simulink model "HighLevel_RaspberryPi"  (R2016a)
settings: Solver=ode3  StartTime=0.0  StopTime=inf  RelTol=1e-3
model workspace (MAT data in the model file):
  neighborhood = [301 101]
  num_pics = 16
undefined symbols (not defined in the file): gray
libraries: simulink x21, dspswit3 x6, visiontextngfix x5, visiontransforms x2, embdlinuxlib x2, visionanalysis x1, visionstatistics x1, visiongeotforms x1
settings Model: SimulationMode=external  ExtModeTrigDuration=100  Creator=Grisha  LastModifiedBy=Ryhor
settings SolverCC: PositivePriorityOrder=on
settings DataIOCC: LimitDataPoints=on  SaveOutput=off  SignalLogging=off  SaveTime=off
settings OptimizationCC: EfficientMapNaN2IntZero=off  OptimizeModelRefInitCode=on  LifeSpan=Inf  MaxStackSize=64
settings DebuggingCC: MultiTaskRateTransMsg=warning  ParameterPrecisionLossMsg=none  AllowSymbolicDim=off  StateNameClashWarn=warning
settings HardwareCC: ProdBitPerPointer=32  ProdLargestAtomicInteger=Long  ProdLargestAtomicFloat=Double  ProdWordSize=32  ProdHWDeviceType=ARM Compatible->ARM Cortex
settings ModelReferenceCC: PropagateSignalLabelsOutOfModel=off
settings RTWCC: SystemTargetFile=ert.tlc  HardwareBoard=Raspberry Pi  TemplateMakefile=ert_default_tmf  GenerateReport=on  RTWVerbose=off  Toolchain=GNU GCC Raspberry Pi  IncludeHyperlinkInReport=on  LaunchReport=on  GenerateTraceInfo=on  GenerateTraceReport=on  GenerateTraceReportSl=on  GenerateTraceReportSf=on  GenerateTraceReportEml=on
settings CodeAppCC: ForceParamTrailComments=on  IgnoreCustomStorageClasses=off  OperatorAnnotations=on  SimulinkDataObjDesc=on  SFDataObjDesc=on  MATLABFcnDesc=on  MangleLength=10  InsertBlockDesc=on  MATLABSourceComments=on
settings ERTTargetCC: SupportVariableSizeSignals=on  ExtMode=on  ExtModeMexArgs='192.168.1.102' 0 17725

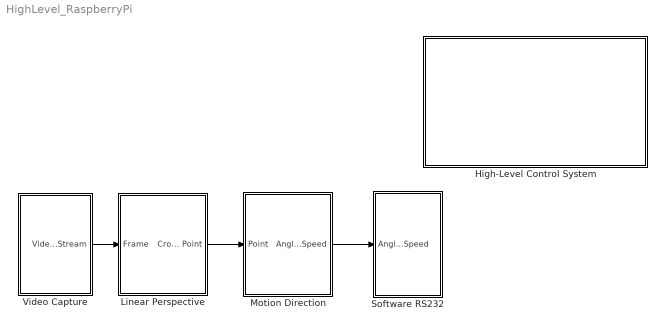
== system HighLevel_RaspberryPi ==
  High-Level Control System : Subsystem
      mask Display: image('C:\Users\Ryhor\Pictures\raspberry-pi-2-primary-100569130-large.png');
  Linear Perspective : Subsystem
  Motion Direction : Subsystem
  Software RS232 : Subsystem
  Video Capture : Subsystem
  wires:
  Motion Direction/1(Angle Speed) -> Software RS232/1(Angle Speed)
  Video Capture/1(Video Stream) -> Linear Perspective/1(Frame)
  Linear Perspective/1(Cross Point) -> Motion Direction/1(Point)

== system HighLevel_RaspberryPi/High-Level Control System ==

== system HighLevel_RaspberryPi/Linear Perspective ==
  Frame : Inport
  Edge Detection : visionanalysis/Edge Detection  method=Roberts  outputType=Binary image  userDefinedThreshold=off  thresholdSource=Input port  threshold=20  thresholdTuning=4  edgeThinning=off  threshold_canny=[0.25 0.60]  autoPercent=90  sigma=1  prodOutputMode=Binary point scaling  prodOutputWordLength=32  prodOutputFracLength=8  roundingMode=Floor  overflowMode=off
  Find Al Lines From HoughTransforms : Subsystem
  Line Sort : Subsystem
  Lines Crossing Points : Subsystem
  Cross Point : Outport
  wires:
  Find Al Lines From HoughTransforms/1(All_Lines) -> Line Sort/2(All Lines)
  Line Sort/2(Desired Line Coord) -> Lines Crossing Points/2(Line Coord)
  Line Sort/1(Image Out) -> Lines Crossing Points/1(Image In)
  Edge Detection/1 -> Find Al Lines From HoughTransforms/1(BW)
  Lines Crossing Points/1(Cross Point) -> Cross Point/1
  Frame/1 -> Find Al Lines From HoughTransforms/2(Grey), Line Sort/1(RGB Image), Edge Detection/1

== system HighLevel_RaspberryPi/Motion Direction ==
  Point : Inport
  Constant : Constant  Value=160  OutDataTypeStr=uint16
  Constant1 : Constant  Value=140  OutDataTypeStr=uint8
  Constant2 : Constant  Value=100  OutDataTypeStr=uint8
  Selector : Selector  NumberOfDimensions=2  InputPortWidth=3  IndexOptions=Index vector (dialog),Index vector (dialog)  Indices=1 ,1  OutputSizes=1,1
  Sum : Sum  Inputs=|+-
  Switch : Switch  Criteria=u2 > Threshold
  Angle Speed : Outport
  wires:
  Constant/1 -> Sum/2
  Constant1/1 -> Switch/1
  Constant2/1 -> Switch/3
  Point/1 -> Selector/1
  Selector/1 -> Sum/1
  Sum/1 -> Switch/2
  Switch/1 -> Angle Speed/1

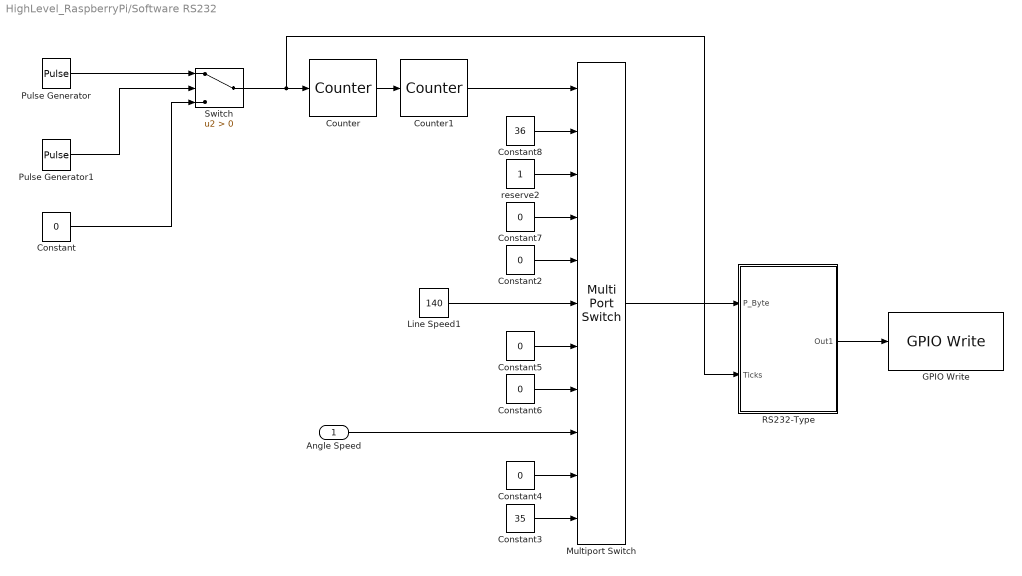
== system HighLevel_RaspberryPi/Software RS232 ==
  Angle Speed : Inport
  Constant : Constant  Value=0  OutDataTypeStr=boolean
  Constant{2,4..7} (5 alike) : Constant  Value=0
  Constant3 : Constant  Value=35
  Constant8 : Constant  Value=36
  Counter : dspswit3/Counter  Direction=Up  CountEvent=Rising edge  CounterSize=User defined  MaxCount=16  InitialCount=1  Output=Hit  HitValue=16  ResetInput=off  SamplesPerFrame=1  Ts=1  CntDtype=double  HitDtype=Logical
  Counter1 : dspswit3/Counter  Direction=Up  CountEvent=Rising edge  CounterSize=User defined  MaxCount=9  InitialCount=0  Output=Count  HitValue=16  ResetInput=off  SamplesPerFrame=1  Ts=1  CntDtype=double  HitDtype=Logical
  GPIO Write : embdlinuxlib/GPIO Write  board=Pi 2 Model B  gpio=14  direction=Output  blockPlatform=Raspberry Pi
  Line Speed1 : Constant  Value=140
  Multiport Switch : MultiPortSwitch  DataPortOrder=Zero-based contiguous  Inputs=10
  Pulse Generator : DiscretePulseGenerator  PulseType=Time based  Period=1/2400  PulseWidth=50  SampleTime=10/57600/16
  Pulse Generator1 : DiscretePulseGenerator  PulseType=Time based  Period=1  PulseWidth=160/2400*100  SampleTime=10/57600/16
  RS232-Type : Subsystem
  Switch : Switch  Criteria=u2 > Threshold
  reserve2 : Constant
  wires:
  Angle Speed/1 -> Multiport Switch/9
  Line Speed1/1 -> Multiport Switch/6
  Constant3/1 -> Multiport Switch/11
  Constant4/1 -> Multiport Switch/10
  Constant6/1 -> Multiport Switch/8
  Constant5/1 -> Multiport Switch/7
  reserve2/1 -> Multiport Switch/3
  Constant8/1 -> Multiport Switch/2
  Constant7/1 -> Multiport Switch/4
  Constant2/1 -> Multiport Switch/5
  Counter/1 -> Counter1/1
  Counter1/1 -> Multiport Switch/1
  Switch/1 -> RS232-Type/2(Ticks), Counter/1
  RS232-Type/1(Out1) -> GPIO Write/1
  Multiport Switch/1 -> RS232-Type/1(P_Byte)
  Pulse Generator/1 -> Switch/1
  Pulse Generator1/1 -> Switch/2
  Constant/1 -> Switch/3

== system HighLevel_RaspberryPi/Video Capture ==
  Rotate : visiongeotforms/Rotate  outSizeR=Expanded to fit rotated input image  src_angle=Specify via dialog  unit_angle=Degrees  angle=pi/2  maxAngle=pi  dispImage=Center  method=Table lookup  fillVal=0  interpMethod=Bilinear  prodOutputMode=Binary point scaling  prodOutputWordLength=32  prodOutputFracLength=10  roundingMode=Nearest  overflowMode=on
  Terminator : Terminator
  Terminator1 : Terminator
  V4L2 Video Capture : embdlinuxlib/V4L2 Video Capture  m_devName='/dev/video0'  roi=[0, 0, 640, 480]  imSizeSelection=320x240  imSize=[640, 480]  pixelFormat=YCbCr 4:2:2  pixelOrder=Planar  sampleTime=1/4  simOutput=Colorbars  blockPlatform=Raspberry Pi
  Video Stream : Outport
  wires:
  V4L2 Video Capture/2 -> Terminator/1
  V4L2 Video Capture/1 -> Rotate/1
  V4L2 Video Capture/3 -> Terminator1/1
  Rotate/1 -> Video Stream/1

== system HighLevel_RaspberryPi/Linear Perspective/Find Al Lines From HoughTransforms ==
  BW : Inport
  Grey : Inport  Port=2
  Constant : Constant  Value=1000
  Find Local Maxima1 : visionstatistics/Find Local Maxima  num_peaks=num_pics  nhood_size=[21 21]  src_thresh=Obsolete9b  src_thresh_inuse=Input port  threshold=1  inputIsHough=on  dt_peak=uint16  isOutVarDim=on  dt_count=uint16
  Find_All_Lines : Subsystem
  Hough Transform : visiontransforms/Hough Transform  theta_res=pi/180  rho_res=1  out_theta_rho=on  outdtmode=double  firstCoeffMode=Binary point scaling  firstCoeffWordLength=16  firstCoeffFracLength=14  secondCoeffMode=Binary point scaling  secondCoeffWordLength=32  secondCoeffFracLength=16  outputMode=Binary point scaling  outputWordLength=16  outputFracLength=0  accumMode=Binary point scaling  accumWordLength=32  accumFracLength=20  prodOutputMode=Binary point scaling  prodOutputWordLength=32  prodOutputFracLength=20  memoryMode=Binary point scaling  memoryWordLength=32  memoryFracLength=16  roundingMode=Nearest  overflowMode=on
  Slider Gain : simulink/Math Operations/Slider Gain  low=0  gain=0.046083  high=1
  All_Lines : Outport
  wires:
  Find Local Maxima1/1 -> Find_All_Lines/1(In1)
  Hough Transform/3 -> Find_All_Lines/3(Rho)
  Find_All_Lines/1(Out1) -> All_Lines/1
  Hough Transform/1 -> Find Local Maxima1/1
  Slider Gain/1 -> Find Local Maxima1/2
  Grey/1 -> Find_All_Lines/4(Grey)
  Constant/1 -> Slider Gain/1
  Hough Transform/2 -> Find_All_Lines/2(Theta)
  BW/1 -> Hough Transform/1

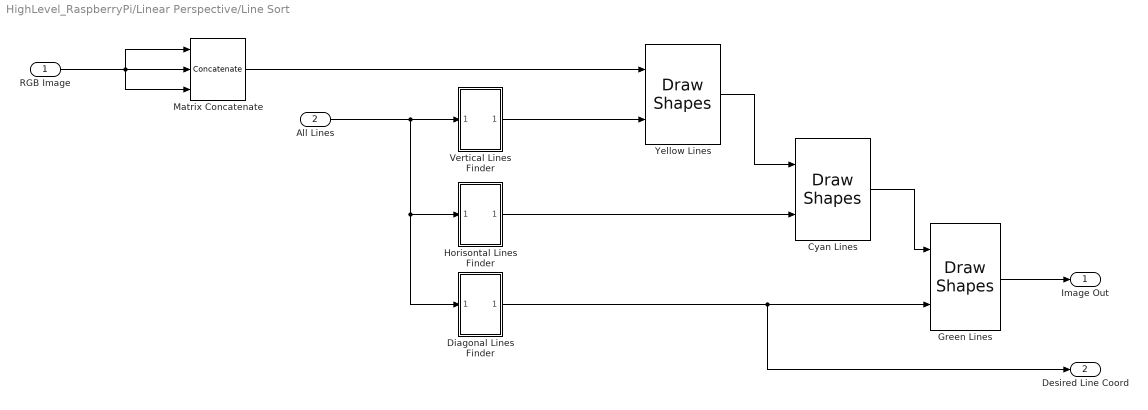
== system HighLevel_RaspberryPi/Linear Perspective/Line Sort ==
  RGB Image : Inport
  All Lines : Inport  Port=2
  Cyan Lines : visiontextngfix/Draw Shapes  shape=Lines  fill=off  lineWidth=2  fillClrSource=Specify via dialog  display=User-specified value  intensity=200  color=[0 100 100]  opacity=0.6  viewport=Entire image  antialiasing=off  inType=Obsolete  imagePorts=One multidimensional signal  prodOutputMode=Binary point scaling  prodOutputWordLength=32  prodOutputFracLength=14  memoryMode=Specify word length  memoryWordLength=16  memoryFracLength=14  roundingMode=Floor  overflowMode=off
  Diagonal Lines Finder : Subsystem
  Green Lines : visiontextngfix/Draw Shapes  shape=Lines  fill=off  lineWidth=1  fillClrSource=Specify via dialog  display=User-specified value  intensity=200  color=[0 255 0]  opacity=0.6  viewport=Entire image  antialiasing=off  inType=Obsolete  imagePorts=One multidimensional signal  prodOutputMode=Binary point scaling  prodOutputWordLength=32  prodOutputFracLength=14  memoryMode=Specify word length  memoryWordLength=16  memoryFracLength=14  roundingMode=Floor  overflowMode=off
  Horisontal Lines Finder : Subsystem
  Matrix Concatenate : Concatenate  NumInputs=3  Mode=Multidimensional array  ConcatenateDimension=3
  Vertical Lines Finder : Subsystem
  Yellow Lines : visiontextngfix/Draw Shapes  shape=Lines  fill=off  lineWidth=2  fillClrSource=Specify via dialog  display=User-specified value  intensity=200  color=[255 255 0]  opacity=0.6  viewport=Entire image  antialiasing=off  inType=Obsolete  imagePorts=One multidimensional signal  prodOutputMode=Binary point scaling  prodOutputWordLength=32  prodOutputFracLength=14  memoryMode=Specify word length  memoryWordLength=16  memoryFracLength=14  roundingMode=Floor  overflowMode=off
  Image Out : Outport
  Desired Line Coord : Outport  Port=2
  wires:
  Vertical Lines Finder/1(Out1) -> Yellow Lines/2
  Cyan Lines/1 -> Green Lines/1
  Diagonal Lines Finder/1(Out2) -> Desired Line Coord/1, Green Lines/2
  Yellow Lines/1 -> Cyan Lines/1
  Horisontal Lines Finder/1(Out1) -> Cyan Lines/2
  Green Lines/1 -> Image Out/1
  All Lines/1 -> Diagonal Lines Finder/1(In1), Horisontal Lines Finder/1(In1), Vertical Lines Finder/1(In1)
  Matrix Concatenate/1 -> Yellow Lines/1
  RGB Image/1 -> Matrix Concatenate/3, Matrix Concatenate/2, Matrix Concatenate/1

== system HighLevel_RaspberryPi/Linear Perspective/Lines Crossing Points ==
  Image In : Inport
  Line Coord : Inport  Port=2
  If : If  IfExpression=u1 > 1
  If Action Subsystem : Subsystem  TreatAsAtomicUnit=on
  If Action Subsystem1 : Subsystem  TreatAsAtomicUnit=on
  Probe : Probe  ProbeWidth=off  ProbeSampleTime=off  ProbeComplexSignal=off  ProbeSignalDimensions=on
  Selector : Selector  NumberOfDimensions=2  InputPortWidth=3  IndexOptions=Index vector (dialog),Index vector (dialog)  Indices=1,1  OutputSizes=1,1
  Switch : Switch  Criteria=u2 > Threshold  Threshold=1
  Video Viewer2 : VideoViewer  colormapValue=gray(256)  FigPos=[716 982 712 582]
  Cross Point : Outport
  wires:
  Probe/1 -> Selector/1
  Selector/1 -> Switch/2, If Action Subsystem/1(In4), If/1
  If/2 -> If Action Subsystem1/Action
  If/1 -> If Action Subsystem/Action
  If Action Subsystem/1(Image Out) -> Switch/1
  If Action Subsystem1/1(Out1) -> Switch/3
  Line Coord/1 -> If Action Subsystem/2(Data Lines), Probe/1
  Image In/1 -> If Action Subsystem1/1(Image In), If Action Subsystem/3(Image In)
  Switch/1 -> Video Viewer2/1
  If Action Subsystem/2(Cross) -> Cross Point/1

== system HighLevel_RaspberryPi/Software RS232/RS232-Type ==
  P_Byte : Inport
  Ticks : Inport  Port=2
  1 + 1+1+ Start Bit : Constant  Value=[1 1 1 0]  OutDataTypeStr=boolean
  Data Type Conv : DataTypeConversion  OutDataTypeStr=boolean
  MATLAB Function : MATLAB Function  TreatAsAtomicUnit=on
  Mux : Mux  Inputs=3
  Parallel-Serial Register 16-1 : Subsystem
  Scope : Scope  NumInputPorts=2
  Stop Bi + 1 + 1 + 1 : Constant  Value=[1 1 1 1]  OutDataTypeStr=boolean
  Out1 : Outport
  wires:
  Parallel-Serial Register 16-1/1(SWord) -> Out1/1, Scope/2
  Mux/1 -> Parallel-Serial Register 16-1/1(P_D_Word)
  Data Type Conv/1 -> Mux/2
  P_Byte/1 -> MATLAB Function/1(u)
  MATLAB Function/1(y) -> Data Type Conv/1
  Ticks/1 -> Scope/1, Parallel-Serial Register 16-1/2(Ticks)
  1 + 1+1+ Start Bit/1 -> Mux/1
  Stop Bi + 1 + 1 + 1/1 -> Mux/3

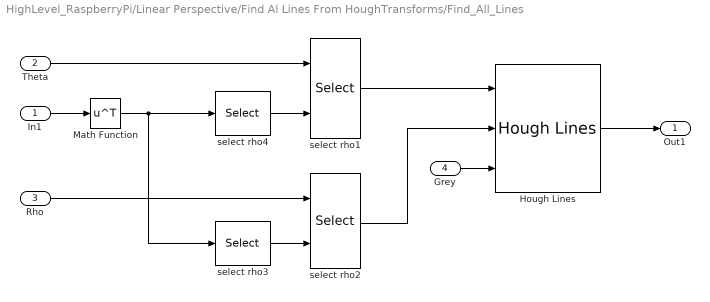
== system HighLevel_RaspberryPi/Linear Perspective/Find Al Lines From HoughTransforms/Find_All_Lines ==
  In1 : Inport
  Theta : Inport  Port=2
  Rho : Inport  Port=3
  Grey : Inport  Port=4
  Hough Lines : visiontransforms/Hough Lines  sineCompMethod=Trigonometric function  thetaRes=pi/180  firstCoeffMode=Specify word length  firstCoeffWordLength=16  firstCoeffFracLength=15  prodOutputMode=Binary point scaling  prodOutputWordLength=32  prodOutputFracLength=16  roundingMode=Nearest  overflowMode=on
  Math Function : Math  Operator=transpose  SaturateOnIntegerOverflow=on
  select rho1 : Selector  NumberOfDimensions=2  InputPortWidth=3  IndexOptions=Select all,Index vector (port)  Indices=1,1  OutputSizes=1,
  select rho2 : Selector  NumberOfDimensions=2  InputPortWidth=3  IndexOptions=Select all,Index vector (port)  Indices=1,1  OutputSizes=1,
  select rho3 : Selector  NumberOfDimensions=2  InputPortWidth=3  IndexOptions=Index vector (dialog),Select all  Indices=2,1  OutputSizes=1,
  select rho4 : Selector  NumberOfDimensions=2  InputPortWidth=3  IndexOptions=Index vector (dialog),Select all  Indices=1,1  OutputSizes=1,
  Out1 : Outport
  wires:
  Theta/1 -> select rho1/1
  Grey/1 -> Hough Lines/3
  In1/1 -> Math Function/1
  select rho2/1 -> Hough Lines/2
  select rho4/1 -> select rho1/2
  select rho3/1 -> select rho2/2
  Rho/1 -> select rho2/1
  Math Function/1 -> select rho3/1, select rho4/1
  Hough Lines/1 -> Out1/1
  select rho1/1 -> Hough Lines/1

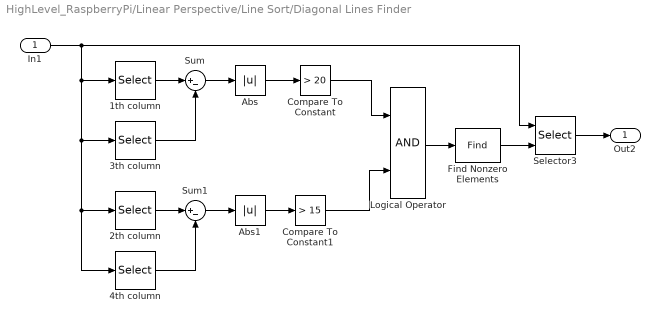
== system HighLevel_RaspberryPi/Linear Perspective/Line Sort/Diagonal Lines Finder ==
  In1 : Inport
  1th column : Selector  NumberOfDimensions=2  InputPortWidth=3  IndexOptions=Select all,Index vector (dialog)  Indices=[1 3],1  OutputSizes=1,1
  2th column : Selector  NumberOfDimensions=2  InputPortWidth=3  IndexOptions=Select all,Index vector (dialog)  Indices=[1 3],2  OutputSizes=1,1
  3th column : Selector  NumberOfDimensions=2  InputPortWidth=3  IndexOptions=Select all,Index vector (dialog)  Indices=[1 3],3  OutputSizes=1,1
  4th column : Selector  NumberOfDimensions=2  InputPortWidth=3  IndexOptions=Select all,Index vector (dialog)  Indices=[1 3],4  OutputSizes=1,1
  Abs : Abs
  Abs1 : Abs
  Compare To Constant : simulink/Logic and Bit Operations/Compare To Constant  relop=>  const=20  OutDataTypeStr=boolean
  Compare To Constant1 : simulink/Logic and Bit Operations/Compare To Constant  relop=>  const=15  OutDataTypeStr=boolean
  Find Nonzero Elements : Find  NumberOfInputDimensions=3
  Logical Operator : Logic  AllPortsSameDT=off  OutDataTypeStr=boolean
  Selector3 : Selector  NumberOfDimensions=2  InputPortWidth=3  IndexOptions=Index vector (port),Select all  Indices=[1 3],3  OutputSizes=1,1
  Sum : Sum  Inputs=|+-
  Sum1 : Sum  Inputs=|+-
  Out2 : Outport
  wires:
  1th column/1 -> Sum/1
  3th column/1 -> Sum/2
  Abs/1 -> Compare To Constant/1
  Sum/1 -> Abs/1
  2th column/1 -> Sum1/1
  4th column/1 -> Sum1/2
  Abs1/1 -> Compare To Constant1/1
  Sum1/1 -> Abs1/1
  Selector3/1 -> Out2/1
  Compare To Constant1/1 -> Logical Operator/2
  In1/1 -> 4th column/1, 2th column/1, 3th column/1, 1th column/1, Selector3/1
  Logical Operator/1 -> Find Nonzero Elements/1
  Compare To Constant/1 -> Logical Operator/1
  Find Nonzero Elements/1 -> Selector3/2

== system HighLevel_RaspberryPi/Linear Perspective/Line Sort/Horisontal Lines Finder ==
  In1 : Inport
  2th column : Selector  NumberOfDimensions=2  InputPortWidth=3  IndexOptions=Select all,Index vector (dialog)  Indices=[1 3],2  OutputSizes=1,1
  4th column : Selector  NumberOfDimensions=2  InputPortWidth=3  IndexOptions=Select all,Index vector (dialog)  Indices=[1 3],4  OutputSizes=1,1
  Abs : Abs
  Compare To Constant : simulink/Logic and Bit Operations/Compare To Constant  relop=<=  const=15  OutDataTypeStr=boolean
  Find Nonzero Elements : Find  NumberOfInputDimensions=3
  Selector3 : Selector  NumberOfDimensions=2  InputPortWidth=3  IndexOptions=Index vector (port),Select all  Indices=[1 3],3  OutputSizes=1,1
  Sum : Sum  Inputs=|+-
  Out1 : Outport
  wires:
  2th column/1 -> Sum/1
  4th column/1 -> Sum/2
  Abs/1 -> Compare To Constant/1
  Sum/1 -> Abs/1
  Selector3/1 -> Out1/1
  Compare To Constant/1 -> Find Nonzero Elements/1
  Find Nonzero Elements/1 -> Selector3/2
  In1/1 -> 4th column/1, 2th column/1, Selector3/1

== system HighLevel_RaspberryPi/Linear Perspective/Line Sort/Vertical Lines Finder ==
  In1 : Inport
  1th column : Selector  NumberOfDimensions=2  InputPortWidth=3  IndexOptions=Select all,Index vector (dialog)  Indices=[1 3],1  OutputSizes=1,1
  3th column : Selector  NumberOfDimensions=2  InputPortWidth=3  IndexOptions=Select all,Index vector (dialog)  Indices=[1 3],3  OutputSizes=1,1
  Abs : Abs
  Compare To Constant : simulink/Logic and Bit Operations/Compare To Constant  relop=<=  const=20  OutDataTypeStr=boolean
  Find Nonzero Elements : Find  NumberOfInputDimensions=3
  Selector3 : Selector  NumberOfDimensions=2  InputPortWidth=3  IndexOptions=Index vector (port),Select all  Indices=[1 3],3  OutputSizes=1,1
  Sum : Sum  Inputs=|+-
  Out1 : Outport
  wires:
  1th column/1 -> Sum/1
  3th column/1 -> Sum/2
  Abs/1 -> Compare To Constant/1
  Sum/1 -> Abs/1
  Selector3/1 -> Out1/1
  Compare To Constant/1 -> Find Nonzero Elements/1
  Find Nonzero Elements/1 -> Selector3/2
  In1/1 -> 3th column/1, 1th column/1, Selector3/1

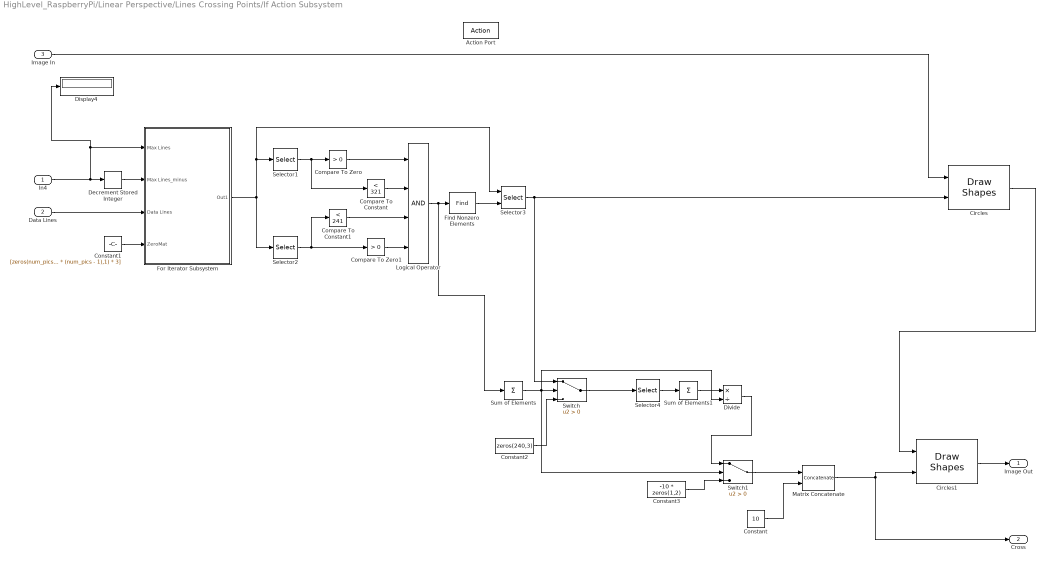
== system HighLevel_RaspberryPi/Linear Perspective/Lines Crossing Points/If Action Subsystem ==
  In4 : Inport
  Data Lines : Inport  Port=2
  Image In : Inport  Port=3
  Action Port : ActionPort  PropagateVarSize=During execution  ActionType=then
  Circles : visiontextngfix/Draw Shapes  shape=Circles  fill=off  lineWidth=2  fillClrSource=Specify via dialog  display=User-specified value  intensity=200  color=[255 0 0]  opacity=0.6  viewport=Entire image  antialiasing=off  inType=Obsolete  imagePorts=One multidimensional signal  prodOutputMode=Binary point scaling  prodOutputWordLength=32  prodOutputFracLength=14  memoryMode=Specify word length  memoryWordLength=16  memoryFracLength=14  roundingMode=Floor  overflowMode=off
  Circles1 : visiontextngfix/Draw Shapes  shape=Circles  fill=off  lineWidth=2  fillClrSource=Specify via dialog  display=User-specified value  intensity=200  color=[200 0 200]  opacity=0.6  viewport=Entire image  antialiasing=off  inType=Obsolete  imagePorts=One multidimensional signal  prodOutputMode=Binary point scaling  prodOutputWordLength=32  prodOutputFracLength=14  memoryMode=Specify word length  memoryWordLength=16  memoryFracLength=14  roundingMode=Floor  overflowMode=off
  Compare To Constant : simulink/Logic and Bit Operations/Compare To Constant  relop=<  const=321  OutDataTypeStr=boolean
  Compare To Constant1 : simulink/Logic and Bit Operations/Compare To Constant  relop=<  const=241  OutDataTypeStr=boolean
  Compare To Zero : simulink/Logic and Bit Operations/Compare To Zero  relop=>  OutDataTypeStr=boolean
  Compare To Zero1 : simulink/Logic and Bit Operations/Compare To Zero  relop=>  OutDataTypeStr=boolean
  Constant : Constant  Value=10  OutDataTypeStr=int32
  Constant1 : Constant  Value=[zeros(num_pics * (num_pics - 1), 2), ones(num_pics * (num_pics - 1),1) * 3]  VectorParams1D=off  OutDataTypeStr=int32
  Constant2 : Constant  Value=zeros(240,3)  VectorParams1D=off  OutDataTypeStr=int32
  Constant3 : Constant  Value=-10 * zeros(1,2)  VectorParams1D=off  OutDataTypeStr=int32
  Decrement Stored Integer : simulink/Additional Math & Discrete/Additional Math: Increment - Decrement/Decrement Stored Integer
  Display4 : Display
  Divide : Product  Inputs=*/
  Find Nonzero Elements : Find  NumberOfInputDimensions=3
  For Iterator Subsystem : Subsystem  TreatAsAtomicUnit=on
  Logical Operator : Logic  Inputs=4  AllPortsSameDT=off  OutDataTypeStr=boolean
  Matrix Concatenate : Concatenate  Mode=Multidimensional array  ConcatenateDimension=2
  Selector1 : Selector  NumberOfDimensions=2  InputPortWidth=3  IndexOptions=Select all,Index vector (dialog)  Indices=[1 3],1  OutputSizes=1,1
  Selector2 : Selector  NumberOfDimensions=2  InputPortWidth=3  IndexOptions=Select all,Index vector (dialog)  Indices=[1 3],2  OutputSizes=1,1
  Selector3 : Selector  NumberOfDimensions=2  InputPortWidth=3  IndexOptions=Index vector (port),Select all  Indices=[1 3],1  OutputSizes=1,1
  Selector4 : Selector  NumberOfDimensions=2  InputPortWidth=3  IndexOptions=Select all,Index vector (dialog)  Indices=[1 3],[1 2]  OutputSizes=1,1
  Sum of Elements : Sum  Inputs=+  AccumDataTypeStr=int32
  Sum of Elements1 : Sum  Inputs=+  CollapseMode=Specified dimension
  Switch : Switch  Criteria=u2 > Threshold
  Switch1 : Switch  Criteria=u2 > Threshold
  Image Out : Outport
  Cross : Outport  Port=2
  wires:
  Find Nonzero Elements/1 -> Selector3/2
  Compare To Zero/1 -> Logical Operator/1
  Compare To Constant1/1 -> Logical Operator/3
  Decrement Stored Integer/1 -> For Iterator Subsystem/2(Max Lines_minus)
  Compare To Constant/1 -> Logical Operator/2
  Selector2/1 -> Compare To Constant1/1, Compare To Zero1/1
  Selector1/1 -> Compare To Zero/1, Compare To Constant/1
  Compare To Zero1/1 -> Logical Operator/4
  For Iterator Subsystem/1(Out1) -> Selector1/1, Selector3/1, Selector2/1
  Logical Operator/1 -> Sum of Elements/1, Find Nonzero Elements/1
  Constant1/1 -> For Iterator Subsystem/4("ZeroMat ")
  In4/1 -> Display4/1, For Iterator Subsystem/1(Max Lines), Decrement Stored Integer/1
  Selector3/1 -> Circles/2, Switch/1
  Data Lines/1 -> For Iterator Subsystem/3(Data Lines)
  Image In/1 -> Circles/1
  Selector4/1 -> Sum of Elements1/1
  Sum of Elements1/1 -> Divide/1
  Divide/1 -> Switch1/1
  Switch/1 -> Selector4/1
  Constant2/1 -> Switch/3
  Constant3/1 -> Switch1/3
  Circles/1 -> Circles1/1
  Matrix Concatenate/1 -> Cross/1, Circles1/2
  Constant/1 -> Matrix Concatenate/2
  Switch1/1 -> Matrix Concatenate/1
  Sum of Elements/1 -> Switch1/2, Divide/2, Switch/2
  Circles1/1 -> Image Out/1

== system HighLevel_RaspberryPi/Linear Perspective/Lines Crossing Points/If Action Subsystem1 ==
  Image In : Inport
  Action Port : ActionPort  ActionType=else
  Out1 : Outport
  wires:
  Image In/1 -> Out1/1

== system HighLevel_RaspberryPi/Software RS232/RS232-Type/Parallel-Serial Register 16-1 ==
  P_D_Word : Inport
  Ticks : Inport  Port=2
  Counter 2^4 : Subsystem
  Demux : Demux  Outputs=8
  Demux1 : Demux  Outputs=8
  High Byte : Selector  InputPortWidth=16  IndexOptions=Index vector (dialog)  Indices=[9:16]  OutputSizes=1
  Low Byte : Selector  InputPortWidth=16  IndexOptions=Index vector (dialog)  Indices=[1:8]  OutputSizes=1
  Multyplexer 8-1 : Subsystem
  Multyplexer 8-2 : Subsystem
  Switch : Switch  Criteria=u2 > Threshold
  SWord : Outport
  wires:
  High Byte/1 -> Demux/1
  Multyplexer 8-2/1(Out1) -> Switch/3
  Multyplexer 8-1/1(Out1) -> Switch/1
  Counter 2^4/1(A) -> Switch/2
  Counter 2^4/2(B) -> Multyplexer 8-2/9(B), Multyplexer 8-1/9(B)
  Counter 2^4/3(C) -> Multyplexer 8-2/10(C), Multyplexer 8-1/10(C)
  Counter 2^4/4(D) -> Multyplexer 8-2/11(D), Multyplexer 8-1/11(D)
  Low Byte/1 -> Demux1/1
  P_D_Word/1 -> Low Byte/1, High Byte/1
  Switch/1 -> SWord/1
  Demux1/4 -> Multyplexer 8-2/4(3b)
  Demux1/3 -> Multyplexer 8-2/3(2b)
  Demux1/5 -> Multyplexer 8-2/5(4b)
  Demux1/6 -> Multyplexer 8-2/6(5b)
  Demux1/2 -> Multyplexer 8-2/2(1b)
  Demux1/1 -> Multyplexer 8-2/1(0b)
  Demux1/7 -> Multyplexer 8-2/7(6b)
  Demux1/8 -> Multyplexer 8-2/8(7b)
  Demux/4 -> Multyplexer 8-1/4(3b)
  Demux/3 -> Multyplexer 8-1/3(2b)
  Demux/5 -> Multyplexer 8-1/5(4b)
  Demux/6 -> Multyplexer 8-1/6(5b)
  Demux/2 -> Multyplexer 8-1/2(1b)
  Demux/1 -> Multyplexer 8-1/1(0b)
  Demux/7 -> Multyplexer 8-1/7(6b)
  Ticks/1 -> Counter 2^4/1(Tick)
  Demux/8 -> Multyplexer 8-1/8(7b)

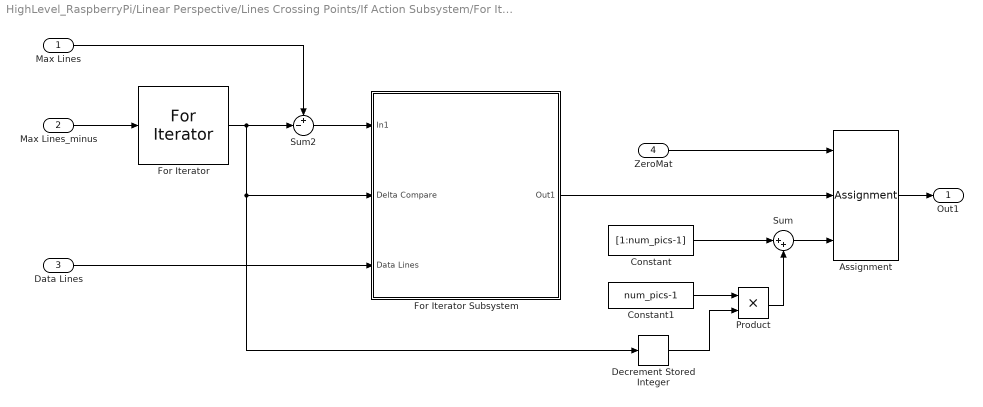
== system HighLevel_RaspberryPi/Linear Perspective/Lines Crossing Points/If Action Subsystem/For Iterator Subsystem ==
  Max Lines : Inport
  Max Lines_minus : Inport  Port=2
  Data Lines : Inport  Port=3
  "ZeroMat " : Inport  Port=4
  Assignment : Assignment  NumberOfDimensions=2  DiagnosticForDimensions=Warning  IndexOptions=Index vector (port),Index vector (dialog)  Indices=1,[1 2]  OutputSizes=1,1
  Constant : Constant  Value=[1:num_pics-1]
  Constant1 : Constant  Value=num_pics-1
  Decrement Stored Integer : simulink/Additional Math & Discrete/Additional Math: Increment - Decrement/Decrement Stored Integer
  For Iterator : ForIterator  IterationSource=external  IterationVariableDataType=int8
  For Iterator Subsystem : Subsystem  TreatAsAtomicUnit=on
  Product : Product
  Sum : Sum  Inputs=|++
  Sum2 : Sum  Inputs=+-|
  Out1 : Outport
  wires:
  Data Lines/1 -> For Iterator Subsystem/3(Data Lines)
  "ZeroMat "/1 -> Assignment/1
  Assignment/1 -> Out1/1
  Constant/1 -> Sum/1
  Max Lines_minus/1 -> For Iterator/1
  Product/1 -> Sum/2
  Sum/1 -> Assignment/3
  For Iterator/1 -> Sum2/2, Decrement Stored Integer/1, For Iterator Subsystem/2(Delta Compare)
  Max Lines/1 -> Sum2/1
  Sum2/1 -> For Iterator Subsystem/1(In1)
  For Iterator Subsystem/1(Out1) -> Assignment/2
  Constant1/1 -> Product/1
  Decrement Stored Integer/1 -> Product/2

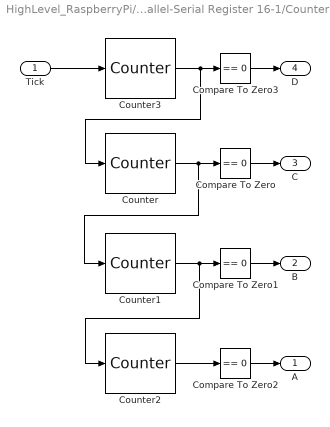
== system HighLevel_RaspberryPi/Software RS232/RS232-Type/Parallel-Serial Register 16-1/Counter 2^4 ==
  Tick : Inport
  Compare To Zero{,1..3} (4 alike) : simulink/Logic and Bit Operations/Compare To Zero  relop===  OutDataTypeStr=boolean
  Counter : dspswit3/Counter  Direction=Up  CountEvent=Rising edge  CounterSize=User defined  MaxCount=1  InitialCount=1  Output=Hit  HitValue=1  ResetInput=off  SamplesPerFrame=1  Ts=1  CntDtype=int8  HitDtype=Boolean
  Counter1 : dspswit3/Counter  Direction=Up  CountEvent=Rising edge  CounterSize=User defined  MaxCount=1  InitialCount=1  Output=Hit  HitValue=1  ResetInput=off  SamplesPerFrame=1  Ts=1  CntDtype=int8  HitDtype=Logical
  Counter2 : dspswit3/Counter  Direction=Up  CountEvent=Rising edge  CounterSize=User defined  MaxCount=1  InitialCount=1  Output=Hit  HitValue=1  ResetInput=off  SamplesPerFrame=1  Ts=1  CntDtype=int8  HitDtype=Logical
  Counter3 : dspswit3/Counter  Direction=Up  CountEvent=Rising edge  CounterSize=User defined  MaxCount=1  InitialCount=1  Output=Hit  HitValue=1  ResetInput=off  SamplesPerFrame=1  Ts=1  CntDtype=int8  HitDtype=Logical
  A : Outport
  B : Outport  Port=2
  C : Outport  Port=3
  D : Outport  Port=4
  wires:
  Tick/1 -> Counter3/1
  Compare To Zero3/1 -> D/1
  Counter3/1 -> Compare To Zero3/1, Counter/1
  Compare To Zero2/1 -> A/1
  Compare To Zero1/1 -> B/1
  Compare To Zero/1 -> C/1
  Counter/1 -> Compare To Zero/1, Counter1/1
  Counter1/1 -> Counter2/1, Compare To Zero1/1
  Counter2/1 -> Compare To Zero2/1

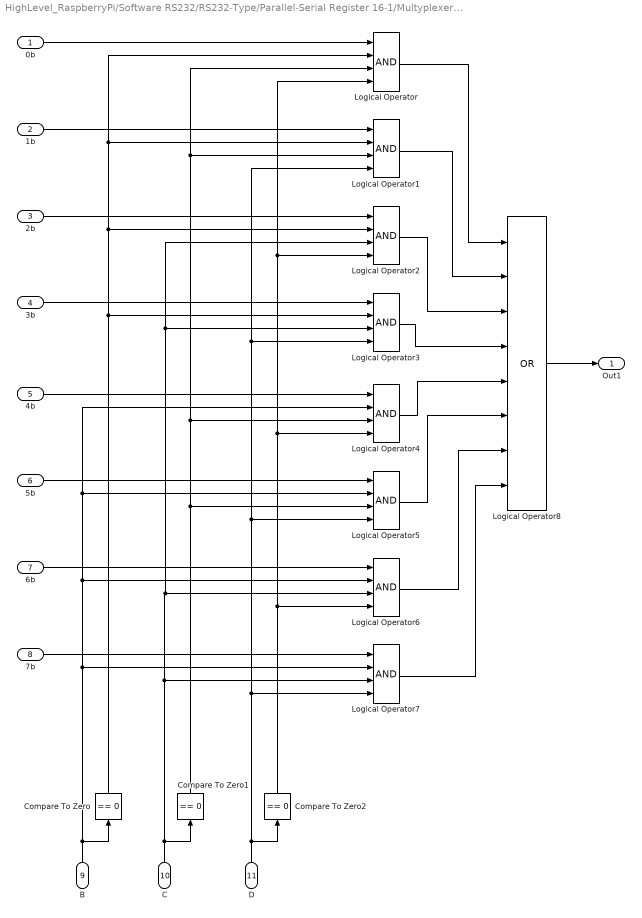
== system HighLevel_RaspberryPi/Software RS232/RS232-Type/Parallel-Serial Register 16-1/Multyplexer 8-1 ==
  0b : Inport
  1b : Inport  Port=2
  2b : Inport  Port=3
  3b : Inport  Port=4
  4b : Inport  Port=5
  5b : Inport  Port=6
  6b : Inport  Port=7
  7b : Inport  Port=8
  B : Inport  Port=9
  C : Inport  Port=10
  D : Inport  Port=11
  Compare To Zero : simulink/Logic and Bit Operations/Compare To Zero  relop===  OutDataTypeStr=boolean
  Compare To Zero1 : simulink/Logic and Bit Operations/Compare To Zero  relop===  OutDataTypeStr=boolean
  Compare To Zero2 : simulink/Logic and Bit Operations/Compare To Zero  relop===  OutDataTypeStr=boolean
  Logical Operator{,1..7} (8 alike) : Logic  Inputs=4  AllPortsSameDT=off  OutDataTypeStr=boolean
  Logical Operator8 : Logic  Operator=OR  Inputs=8  AllPortsSameDT=off  OutDataTypeStr=boolean
  Out1 : Outport
  wires:
  Compare To Zero2/1 -> Logical Operator2/4, Logical Operator/4, Logical Operator4/4, Logical Operator6/4
  D/1 -> Compare To Zero2/1, Logical Operator1/4, Logical Operator3/4, Logical Operator5/4, Logical Operator7/4
  Compare To Zero1/1 -> Logical Operator4/3, Logical Operator1/3, Logical Operator/3, Logical Operator5/3
  C/1 -> Compare To Zero1/1, Logical Operator7/3, Logical Operator6/3, Logical Operator2/3, Logical Operator3/3
  Compare To Zero/1 -> Logical Operator2/2, Logical Operator/2, Logical Operator1/2, Logical Operator3/2
  B/1 -> Compare To Zero/1, Logical Operator4/2, Logical Operator5/2, Logical Operator6/2, Logical Operator7/2
  Logical Operator8/1 -> Out1/1
  5b/1 -> Logical Operator5/1
  6b/1 -> Logical Operator6/1
  7b/1 -> Logical Operator7/1
  4b/1 -> Logical Operator4/1
  3b/1 -> Logical Operator3/1
  2b/1 -> Logical Operator2/1
  1b/1 -> Logical Operator1/1
  0b/1 -> Logical Operator/1
  Logical Operator7/1 -> Logical Operator8/8
  Logical Operator6/1 -> Logical Operator8/7
  Logical Operator5/1 -> Logical Operator8/6
  Logical Operator4/1 -> Logical Operator8/5
  Logical Operator3/1 -> Logical Operator8/4
  Logical Operator2/1 -> Logical Operator8/3
  Logical Operator1/1 -> Logical Operator8/2
  Logical Operator/1 -> Logical Operator8/1

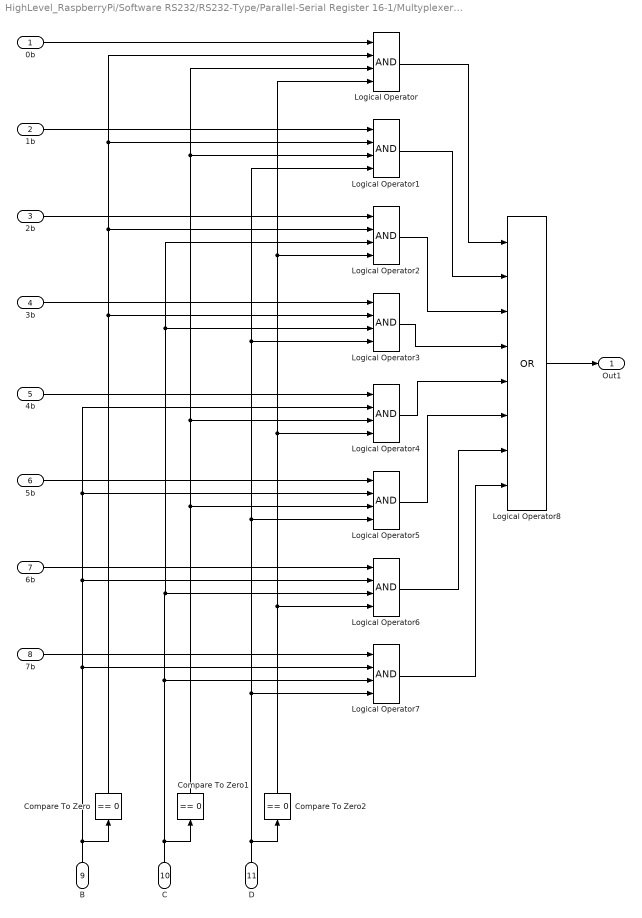
== system HighLevel_RaspberryPi/Software RS232/RS232-Type/Parallel-Serial Register 16-1/Multyplexer 8-2 ==
  0b : Inport
  1b : Inport  Port=2
  2b : Inport  Port=3
  3b : Inport  Port=4
  4b : Inport  Port=5
  5b : Inport  Port=6
  6b : Inport  Port=7
  7b : Inport  Port=8
  B : Inport  Port=9
  C : Inport  Port=10
  D : Inport  Port=11
  Compare To Zero : simulink/Logic and Bit Operations/Compare To Zero  relop===  OutDataTypeStr=boolean
  Compare To Zero1 : simulink/Logic and Bit Operations/Compare To Zero  relop===  OutDataTypeStr=boolean
  Compare To Zero2 : simulink/Logic and Bit Operations/Compare To Zero  relop===  OutDataTypeStr=boolean
  Logical Operator{,1..7} (8 alike) : Logic  Inputs=4  AllPortsSameDT=off  OutDataTypeStr=boolean
  Logical Operator8 : Logic  Operator=OR  Inputs=8  AllPortsSameDT=off  OutDataTypeStr=boolean
  Out1 : Outport
  wires:
  Compare To Zero2/1 -> Logical Operator2/4, Logical Operator/4, Logical Operator4/4, Logical Operator6/4
  D/1 -> Compare To Zero2/1, Logical Operator1/4, Logical Operator3/4, Logical Operator5/4, Logical Operator7/4
  Compare To Zero1/1 -> Logical Operator4/3, Logical Operator1/3, Logical Operator/3, Logical Operator5/3
  C/1 -> Compare To Zero1/1, Logical Operator7/3, Logical Operator6/3, Logical Operator2/3, Logical Operator3/3
  Compare To Zero/1 -> Logical Operator2/2, Logical Operator/2, Logical Operator1/2, Logical Operator3/2
  B/1 -> Compare To Zero/1, Logical Operator4/2, Logical Operator5/2, Logical Operator6/2, Logical Operator7/2
  Logical Operator8/1 -> Out1/1
  5b/1 -> Logical Operator5/1
  6b/1 -> Logical Operator6/1
  7b/1 -> Logical Operator7/1
  4b/1 -> Logical Operator4/1
  3b/1 -> Logical Operator3/1
  2b/1 -> Logical Operator2/1
  1b/1 -> Logical Operator1/1
  0b/1 -> Logical Operator/1
  Logical Operator7/1 -> Logical Operator8/8
  Logical Operator6/1 -> Logical Operator8/7
  Logical Operator5/1 -> Logical Operator8/6
  Logical Operator4/1 -> Logical Operator8/5
  Logical Operator3/1 -> Logical Operator8/4
  Logical Operator2/1 -> Logical Operator8/3
  Logical Operator1/1 -> Logical Operator8/2
  Logical Operator/1 -> Logical Operator8/1

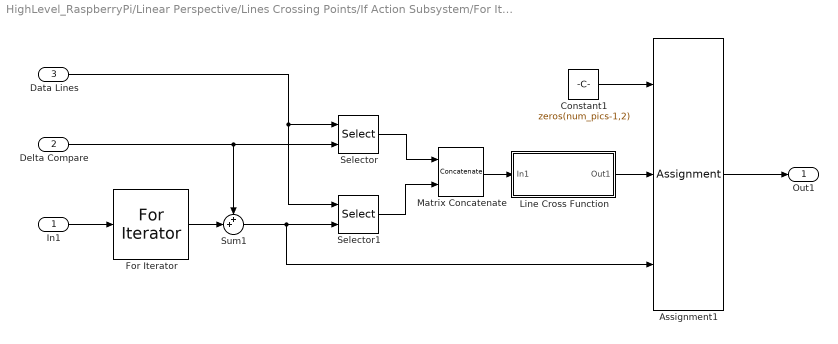
== system HighLevel_RaspberryPi/Linear Perspective/Lines Crossing Points/If Action Subsystem/For Iterator Subsystem/For Iterator Subsystem ==
  In1 : Inport
  Delta Compare : Inport  Port=2
  Data Lines : Inport  Port=3
  Assignment1 : Assignment  NumberOfDimensions=2  DiagnosticForDimensions=Warning  IndexOptions=Index vector (port),Index vector (dialog)  Indices=1,[1 2]  OutputSizes=1,1
  Constant1 : Constant  Value=zeros(num_pics-1,2)  OutDataTypeStr=int32
  For Iterator : ForIterator  IterationSource=external  IterationVariableDataType=int8
  Line Cross Function : Subsystem
  Matrix Concatenate : Concatenate  Mode=Multidimensional array
  Selector : Selector  NumberOfDimensions=2  InputPortWidth=3  IndexOptions=Index vector (port),Select all  Indices=[1 3],1  OutputSizes=1,1
  Selector1 : Selector  NumberOfDimensions=2  InputPortWidth=3  IndexOptions=Index vector (port),Select all  Indices=[1 3],1  OutputSizes=1,1
  Sum1 : Sum  Inputs=++|
  Out1 : Outport
  wires:
  Data Lines/1 -> Selector1/1, Selector/1
  Selector/1 -> Matrix Concatenate/1
  Selector1/1 -> Matrix Concatenate/2
  Matrix Concatenate/1 -> Line Cross Function/1(In1)
  Line Cross Function/1(Out1) -> Assignment1/2
  Constant1/1 -> Assignment1/1
  Sum1/1 -> Assignment1/3, Selector1/2
  Assignment1/1 -> Out1/1
  In1/1 -> For Iterator/1
  For Iterator/1 -> Sum1/2
  Delta Compare/1 -> Selector/2, Sum1/1

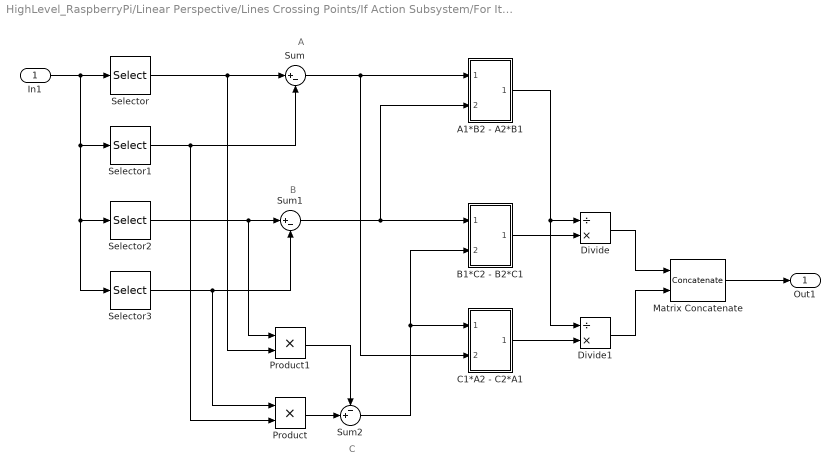
== system HighLevel_RaspberryPi/Linear Perspective/Lines Crossing Points/If Action Subsystem/For Iterator Subsystem/For Iterator Subsystem/Line Cross Function ==
  note: C
  note: B
  note: A
  In1 : Inport
  A1*B2 - A2*B1 : Subsystem
  B1*C2 - B2*C1 : Subsystem
  C1*A2 - C2*A1 : Subsystem
  Divide : Product  Inputs=/*
  Divide1 : Product  Inputs=/*
  Matrix Concatenate : Concatenate  Mode=Multidimensional array  ConcatenateDimension=2
  Product : Product
  Product1 : Product
  Selector : Selector  NumberOfDimensions=2  InputPortWidth=3  IndexOptions=Select all,Index vector (dialog)  Indices=[1 3],2  OutputSizes=1,1
  Selector1 : Selector  NumberOfDimensions=2  InputPortWidth=3  IndexOptions=Select all,Index vector (dialog)  Indices=[1 3],4  OutputSizes=1,1
  Selector2 : Selector  NumberOfDimensions=2  InputPortWidth=3  IndexOptions=Select all,Index vector (dialog)  Indices=[1 3],3  OutputSizes=1,1
  Selector3 : Selector  NumberOfDimensions=2  InputPortWidth=3  IndexOptions=Select all,Index vector (dialog)  Indices=[1 3],1  OutputSizes=1,1
  Sum : Sum  Inputs=|+-
  Sum1 : Sum  Inputs=|+-
  Sum2 : Sum  Inputs=-+|  AccumDataTypeStr=int32  OutDataTypeStr=int32
  Out1 : Outport
  wires:
  Selector/1 -> Sum/1, Product1/2
  Selector1/1 -> Product/2, Sum/2
  In1/1 -> Selector/1, Selector3/1, Selector2/1, Selector1/1
  Selector2/1 -> Product1/1, Sum1/1
  Selector3/1 -> Product/1, Sum1/2
  Product/1 -> Sum2/2
  Product1/1 -> Sum2/1
  Sum/1 -> C1*A2 - C2*A1/2(In2), A1*B2 - A2*B1/1(In1)
  Sum1/1 -> B1*C2 - B2*C1/1(In1), A1*B2 - A2*B1/2(In2)
  Sum2/1 -> C1*A2 - C2*A1/1(In1), B1*C2 - B2*C1/2(In2)
  B1*C2 - B2*C1/1(Out1) -> Divide/2
  A1*B2 - A2*B1/1(Out1) -> Divide1/1, Divide/1
  C1*A2 - C2*A1/1(Out1) -> Divide1/2
  Divide1/1 -> Matrix Concatenate/2
  Divide/1 -> Matrix Concatenate/1
  Matrix Concatenate/1 -> Out1/1

== system HighLevel_RaspberryPi/Linear Perspective/Lines Crossing Points/If Action Subsystem/For Iterator Subsystem/For Iterator Subsystem/Line Cross Function/A1*B2 - A2*B1 ==
  In1 : Inport
  In2 : Inport  Port=2
  Dot Product : DotProduct  OutDataTypeStr=int32  InputSameDT=on
  Dot Product1 : DotProduct  OutDataTypeStr=int32  InputSameDT=on
  Selector4 : Selector  NumberOfDimensions=2  InputPortWidth=3  IndexOptions=Index vector (dialog),Index vector (dialog)  Indices=1,1  OutputSizes=1,1
  Selector5 : Selector  NumberOfDimensions=2  InputPortWidth=3  IndexOptions=Index vector (dialog),Index vector (dialog)  Indices=2,1  OutputSizes=1,1
  Selector6 : Selector  NumberOfDimensions=2  InputPortWidth=3  IndexOptions=Index vector (dialog),Index vector (dialog)  Indices=1,1  OutputSizes=1,1
  Selector7 : Selector  NumberOfDimensions=2  InputPortWidth=3  IndexOptions=Index vector (dialog),Index vector (dialog)  Indices=2,1  OutputSizes=1,1
  Sum3 : Sum  Inputs=|+-
  Out1 : Outport
  wires:
  Dot Product1/1 -> Sum3/2
  Dot Product/1 -> Sum3/1
  Selector6/1 -> Dot Product1/2
  Selector4/1 -> Dot Product/1
  Selector7/1 -> Dot Product1/1
  In1/1 -> Selector7/1, Selector4/1
  In2/1 -> Selector6/1, Selector5/1
  Selector5/1 -> Dot Product/2
  Sum3/1 -> Out1/1

== system HighLevel_RaspberryPi/Linear Perspective/Lines Crossing Points/If Action Subsystem/For Iterator Subsystem/For Iterator Subsystem/Line Cross Function/B1*C2 - B2*C1 ==
  In1 : Inport
  In2 : Inport  Port=2
  Dot Product : DotProduct  OutDataTypeStr=int32  InputSameDT=on
  Dot Product1 : DotProduct  OutDataTypeStr=int32  InputSameDT=on
  Selector4 : Selector  NumberOfDimensions=2  InputPortWidth=3  IndexOptions=Index vector (dialog),Index vector (dialog)  Indices=1,1  OutputSizes=1,1
  Selector5 : Selector  NumberOfDimensions=2  InputPortWidth=3  IndexOptions=Index vector (dialog),Index vector (dialog)  Indices=2,1  OutputSizes=1,1
  Selector6 : Selector  NumberOfDimensions=2  InputPortWidth=3  IndexOptions=Index vector (dialog),Index vector (dialog)  Indices=1,1  OutputSizes=1,1
  Selector7 : Selector  NumberOfDimensions=2  InputPortWidth=3  IndexOptions=Index vector (dialog),Index vector (dialog)  Indices=2,1  OutputSizes=1,1
  Sum3 : Sum  Inputs=|+-
  Out1 : Outport
  wires:
  Dot Product1/1 -> Sum3/2
  Dot Product/1 -> Sum3/1
  Selector6/1 -> Dot Product1/2
  Selector4/1 -> Dot Product/1
  Selector7/1 -> Dot Product1/1
  In1/1 -> Selector7/1, Selector4/1
  In2/1 -> Selector6/1, Selector5/1
  Selector5/1 -> Dot Product/2
  Sum3/1 -> Out1/1

== system HighLevel_RaspberryPi/Linear Perspective/Lines Crossing Points/If Action Subsystem/For Iterator Subsystem/For Iterator Subsystem/Line Cross Function/C1*A2 - C2*A1 ==
  In1 : Inport
  In2 : Inport  Port=2
  Dot Product : DotProduct  OutDataTypeStr=int32  InputSameDT=on
  Dot Product1 : DotProduct  OutDataTypeStr=int32  InputSameDT=on
  Selector4 : Selector  NumberOfDimensions=2  InputPortWidth=3  IndexOptions=Index vector (dialog),Index vector (dialog)  Indices=1,1  OutputSizes=1,1
  Selector5 : Selector  NumberOfDimensions=2  InputPortWidth=3  IndexOptions=Index vector (dialog),Index vector (dialog)  Indices=2,1  OutputSizes=1,1
  Selector6 : Selector  NumberOfDimensions=2  InputPortWidth=3  IndexOptions=Index vector (dialog),Index vector (dialog)  Indices=1,1  OutputSizes=1,1
  Selector7 : Selector  NumberOfDimensions=2  InputPortWidth=3  IndexOptions=Index vector (dialog),Index vector (dialog)  Indices=2,1  OutputSizes=1,1
  Sum3 : Sum  Inputs=|+-
  Out1 : Outport
  wires:
  Dot Product1/1 -> Sum3/2
  Dot Product/1 -> Sum3/1
  Selector6/1 -> Dot Product1/2
  Selector4/1 -> Dot Product/1
  Selector7/1 -> Dot Product1/1
  In1/1 -> Selector7/1, Selector4/1
  In2/1 -> Selector6/1, Selector5/1
  Selector5/1 -> Dot Product/2
  Sum3/1 -> Out1/1

== matlab function HighLevel_RaspberryPi/Software RS232/RS232-Type/MATLAB Function ==
  data: u input; y output
function y = fcn(u)
%#codegen
temp = dec2bin(u,8);
y = zeros(1,8);
for ii = 1: 8
    y(ii) = strcmp(temp(ii),'1');
end
y = fliplr(y);
